simulink model "Spurerkennung"  (R2017a)
settings: Solver=FixedStepDiscrete  StartTime=0.0  StopTime=inf  FixedStep=1/25  RelTol=1e-3  EnableMultiTasking=on
libraries: dspmtrx3 x6, visionanalysis x5, dspvision x2, visionconversions x2, visionsources x1, visionsinks x1
settings Model: NumberOfSteps=5  Creator=Christoph  LastModifiedBy=Christoph
settings SolverCC: EnableConcurrentExecution=on  ConcurrentTasks=on  PositivePriorityOrder=on
settings OptimizationCC: PassReuseOutputArgsAs=Individual arguments  MaxStackSize=64
settings DebuggingCC: ParameterTunabilityLossMsg=error
settings HardwareCC: ProdBitPerPointer=32  ProdBitPerSizeT=32  ProdBitPerPtrDiffT=32  ProdLargestAtomicInteger=Long  ProdLargestAtomicFloat=Double  ProdWordSize=32  ProdHWDeviceType=ARM Compatible->ARM Cortex
settings SFSimCC: MATLABDynamicMemAlloc=off
settings RTWCC: SystemTargetFile=ert.tlc  HardwareBoard=Raspberry Pi  TLCOptions="-aInlineSetEventsForThisBaseRateFcn=TLC_FALSE -aSuppressMultiTaskScheduler=TLC_FALSE  -aRateBasedStepFcn=0"  TemplateMakefile=ert_default_tmf  Description=Embedded Coder  GenerateReport=on  Toolchain=GNU GCC Raspberry Pi  IncludeHyperlinkInReport=on  LaunchReport=on  GenerateTraceInfo=on  GenerateTraceReport=on  GenerateTraceReportSl=on  GenerateTraceReportSf=on  GenerateTraceReportEml=on
settings CodeAppCC: ForceParamTrailComments=on  IgnoreCustomStorageClasses=off  OperatorAnnotations=on  SimulinkDataObjDesc=on  SFDataObjDesc=on  MATLABFcnDesc=on  InsertBlockDesc=on  MATLABSourceComments=on
settings ERTTargetCC: SupportVariableSizeSignals=on

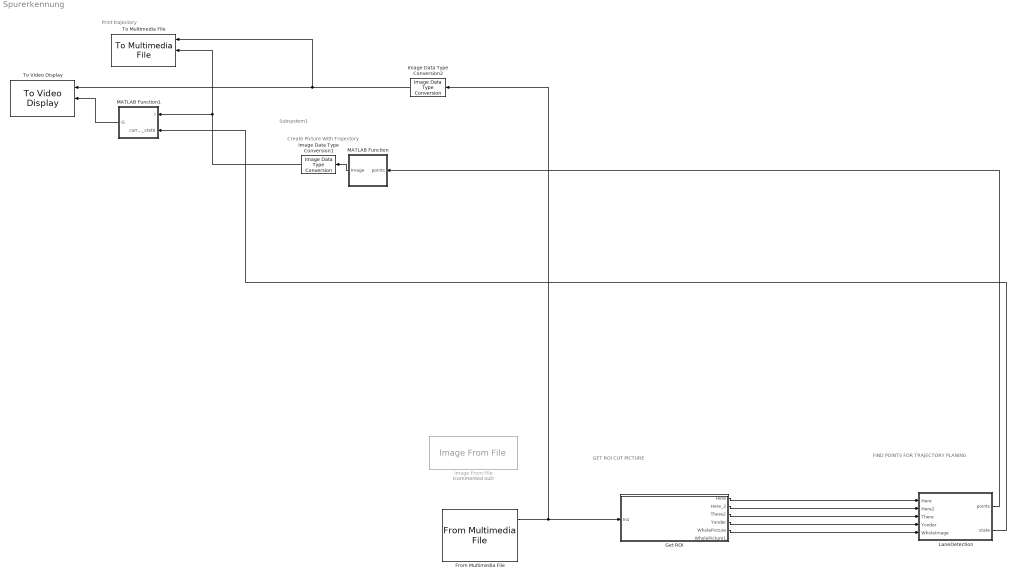
== system Spurerkennung ==
  note: Subsystem1
  note: FIND POINTS FOR TRAJECTORY PLANING
  note: Print trajectory
  note: GET ROI CUT PICTURE
  note: Create Picture With Trajectory
  From Multimedia File : dspvision/From Multimedia File  inputFilename=/Users/Christoph/Documents/workspace/Spurerkennung/Videos/Kreuzung.avi  loop=on  numPlays=inf  outputStreams=Video only  videoDataType=Inherit from file  audioDataType=int16  inheritSampleTime=off  userDefinedSampleTime=1/25  noAudioOutput=off  isIntensityVideo=off  fourcc=RGB  colorVideoFormat=Separate color signals  outputEOF=off  dataOrg=Column-major  audioFrameSize=1024  computeAudioFrameSize=off  outSamplingMode=Sample based
      settings: SourceProductBaseCode=VP
  "Get ROI " : Subsystem
  Image Data Type Conversion1 : visionconversions/Image Data Type Conversion  outDT=single  isSigned=on  wordLen=16  numFracBits=0
      settings: SourceProductName=Computer Vision System Toolbox  SourceProductBaseCode=VP
  Image Data Type Conversion2 : visionconversions/Image Data Type Conversion  outDT=single  isSigned=on  wordLen=16  numFracBits=0
      settings: SourceProductName=Computer Vision System Toolbox  SourceProductBaseCode=VP
  Image From File : visionsources/Image From File  Tag=vipblks_nd  Commented=on  FileName=peppers.png  imagePorts=One multidimensional signal  Ts=inf  ImageDataType=Inherit from input image  Signed=on  WordLength=16  sdImageDataType=uint(8)  FractionLengthMode=User-defined  FractionLength=15  OutPortLabels=R|G|B
      settings: SourceProductName=Computer Vision System Toolbox
  LaneDetection : MATLAB Function  TreatAsAtomicUnit=on
  MATLAB Function : MATLAB Function  TreatAsAtomicUnit=on
  MATLAB Function1 : MATLAB Function  TreatAsAtomicUnit=on
  To Multimedia File : dspvision/To Multimedia File  outputFilename=output.avi  streamSelection=Video only  videoCompressor=None (uncompressed)  audioCompressor=None (uncompressed)  imagePorts=Separate color signals  fileType=AVI  audioDatatype=Determine from input data type  fourcc=RGB  videoQuality=75  mj2000CompFactor=10
      settings: SourceProductName=Computer Vision System Toolbox  SourceProductBaseCode=VP
  To Video Display : visionsinks/To Video Display  windowSizeMode=True size (1:1)  openAtMdlStart=on  fullScreen=off  videoWindowX=547  videoWindowY=164  saveWindowSize=off  videoWindowWidth=640  videoWindowHeight=480  inputColorFormat=RGB  inputType=Obsolete  imagePorts=Separate color signals  OutputDevice=On-screen video monitor  dataOrg=Column-major  isWindowOpen=off
      settings: SourceProductName=Computer Vision System Toolbox
  wires:
  "Get ROI "/1(Here) -> LaneDetection/1(Here)
  "Get ROI "/4(Yonder) -> LaneDetection/4(Yonder)
  Image Data Type Conversion1/1 -> MATLAB Function1/1(I), To Multimedia File/2
  "Get ROI "/3(There2) -> LaneDetection/3(There)
  "Get ROI "/2(Here_2) -> LaneDetection/2(Here2)
  MATLAB Function/1(Image) -> Image Data Type Conversion1/1
  "Get ROI "/5(WholePicture) -> LaneDetection/5(WholeImage)
  Image Data Type Conversion2/1 -> To Multimedia File/1, To Video Display/1
  LaneDetection/1(points) -> MATLAB Function/1(points)
  LaneDetection/2(state) -> MATLAB Function1/2(current_state)
  MATLAB Function1/1(G) -> To Video Display/2
  From Multimedia File/1 -> Image Data Type Conversion2/1, "Get ROI "/1(In1)

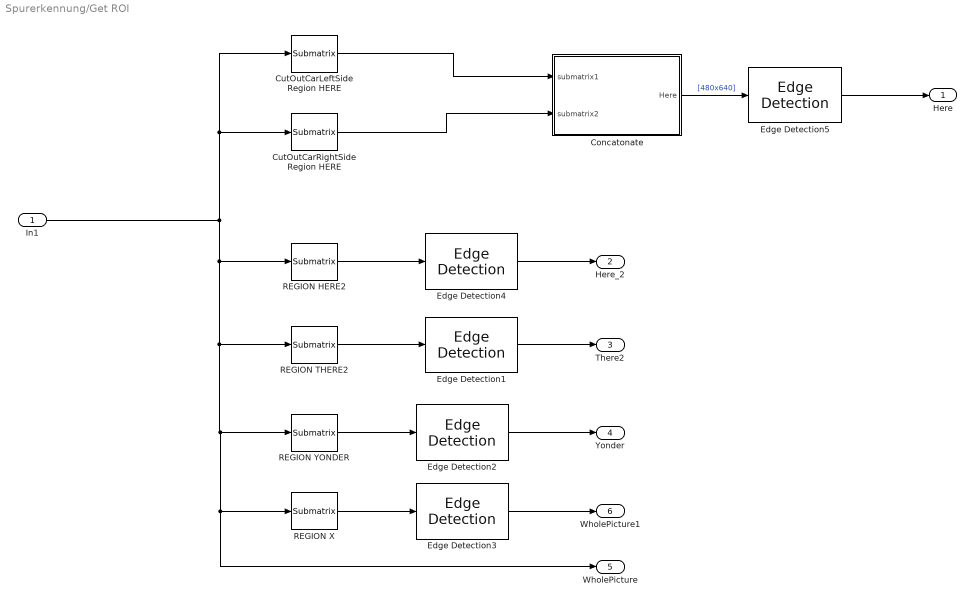
== system Spurerkennung/Get ROI  ==
  In1 : Inport
  Concatonate : MATLAB Function  TreatAsAtomicUnit=on
  CutOutCarLeftSide Region HERE : dspmtrx3/Submatrix  RowSpan=Range of rows  RowStartMode=Index  RowStartIndex=475  RowEndMode=Index  RowEndIndex=480  ColSpan=Range of columns  ColStartMode=Index  ColStartIndex=1  ColEndMode=Index  ColEndIndex=140
  CutOutCarRightSide Region HERE : dspmtrx3/Submatrix  RowSpan=Range of rows  RowStartMode=Index  RowStartIndex=475  RowEndMode=Index  RowEndIndex=480  ColSpan=Range of columns  ColStartMode=Index  ColStartIndex=490  ColEndMode=Last  ColEndIndex=640
  Edge Detection{1..5} (5 alike) : visionanalysis/Edge Detection  method=Sobel  outputType=Binary image  userDefinedThreshold=on  thresholdSource=Specify via dialog  threshold=25  thresholdTuning=4  edgeThinning=off  threshold_canny=[0.1 0.60]  autoPercent=70  sigma=1  prodOutputMode=Binary point scaling  prodOutputWordLength=16  prodOutputFracLength=0  roundingMode=Floor  overflowMode=off
      settings: SourceProductName=Computer Vision System Toolbox  SourceProductBaseCode=VP
  REGION HERE2 : dspmtrx3/Submatrix  RowSpan=Range of rows  RowStartMode=Index  RowStartIndex=330  RowEndMode=Index  RowEndIndex=335  ColSpan=Range of columns  ColStartMode=First  ColStartIndex=1  ColEndMode=Last  ColEndIndex=1
  REGION THERE2 : dspmtrx3/Submatrix  RowSpan=Range of rows  RowStartMode=Index  RowStartIndex=205  RowEndMode=Index  RowEndIndex=210  ColSpan=Range of columns  ColStartMode=First  ColStartIndex=1  ColEndMode=Last  ColEndIndex=1
  REGION X : dspmtrx3/Submatrix  RowSpan=Range of rows  RowStartMode=Index  RowStartIndex=130  RowEndMode=Index  RowEndIndex=135  ColSpan=Range of columns  ColStartMode=First  ColStartIndex=1  ColEndMode=Last  ColEndIndex=1
  REGION YONDER : dspmtrx3/Submatrix  RowSpan=Range of rows  RowStartMode=Index  RowStartIndex=170  RowEndMode=Index  RowEndIndex=175  ColSpan=Range of columns  ColStartMode=First  ColStartIndex=1  ColEndMode=Last  ColEndIndex=1
  Here : Outport
  Here_2 : Outport  Port=2
  There2 : Outport  Port=3
  Yonder : Outport  Port=4
  WholePicture : Outport  Port=5
  WholePicture1 : Outport  Port=6
  wires:
  CutOutCarLeftSide Region HERE/1 -> Concatonate/1(submatrix1)
  In1/1 -> REGION X/1, WholePicture/1, REGION YONDER/1, REGION THERE2/1, REGION HERE2/1, CutOutCarRightSide Region HERE/1, CutOutCarLeftSide Region HERE/1
  CutOutCarRightSide Region HERE/1 -> Concatonate/2(submatrix2)
  REGION HERE2/1 -> Edge Detection4/1
  Edge Detection4/1 -> Here_2/1
  REGION THERE2/1 -> Edge Detection1/1
  Edge Detection1/1 -> There2/1
  REGION YONDER/1 -> Edge Detection2/1
  Edge Detection5/1 -> Here/1
  Concatonate/1(Here) -> Edge Detection5/1  "[480x640]"
  Edge Detection2/1 -> Yonder/1
  REGION X/1 -> Edge Detection3/1
  Edge Detection3/1 -> WholePicture1/1

== matlab function Spurerkennung/MATLAB Function1 ==
  data: I input; G output; current_state input
function G = fcn(I, current_state)

if current_state == 1
    string = 'NORMAL';  
elseif current_state == 2
    string = 'CROSSWALK';  
elseif current_state == 3
    string = 'JUNCTION';

else
    string = 'Normal';
end
    RGB = insertText(I,[1 1],string,'FontSize',18);
G = RGB(:,:,2);

== matlab function Spurerkennung/MATLAB Function ==
  data: Image output; points input
function Image = fcn(points)

%Create picture not necessary if no visualization needed
%TrajectoryImage = zeros(480, 640);

REGIONS_BEGIN = [475 330 205 170];

Image = zeros(480, 640);


for i = 1:size(REGIONS_BEGIN,2)
    Image(REGIONS_BEGIN(i)+2,:) = 1;
end

% 
% p = polyfit(points(1,:), points(2,:), 1);
% x1 = points(1,1);
% x2 = points(1,end);
% x = linspace(x1, x2);
% f = polyval(p,x);
% 
% length_x = size(x,2);
% for j = 1:length_x
%     x_1 = round(x(j));
%     y_1 = round(f(j));
%     if( x_1 >0 && y_1 > 0  && y_1 < 480)
%         Image(y_1, x_1) = 1;
%     end
% end



%disp(points)

lenght = size(points, 2);
% hold off
for i=1:lenght-1
    x1 = points(1,i);
    x2 = points(1,i+1);
    y1 = points(2,i);
    y2 = points(2,i+1);
    p = polyfit([x1 x2], [y1 y2], 1);
%     if(x1 < x2)
%         x2 = 640;
%     else
%         x2 = x2 - 100;
%     end
%     
    x = linspace(x1, x2);
    f = polyval(p, x);
    
    
    length_x = size(x,2);
    for j = 1:length_x
        x_1 = round(x(j));
        y_1 = round(f(j));
        if( x_1 >0 && y_1 > 0  && y_1 < 480)
        Image(y_1, x_1) = 1;
        end
    end
        
        
end

== matlab function Spurerkennung/LaneDetection ==
  data: Here input; Here2 input; There input; Yonder input; WholeImage input; points output; state output

%%%%%%%%% MAIN %%%%%%%%%%%%%%%%%%%%%%%%%%%%%%%%%%%%%%%%%
function [points, state] = fcn(Here, Here2, There, Yonder, WholeImage)

persistent variables
persistent states
persistent initialized
REGIONS = zeros([size(Here) 4]);
REGIONS(:,:,1) = Here;
REGIONS(:,:,2) = Here2;
REGIONS(:,:,3) = There;
REGIONS(:,:,4) = Yonder;

%%%%%%%%%%%%% INIT %%%%%%%%%%%%%%%%%
if(isempty(initialized))
    [variables, states, initialized] = init();
end

%%%%%%%%%%% Sample input %%%%%%%%%%%%%%%%%%%
[all_points, number_of_points]  = FindPointsInLinesAll(variables, REGIONS, true, true);

%%%%%%%%%%%% State machine %%%%%%%%%%%%%%%%%%
[all_points, variables] = RunStateMachine(all_points, number_of_points, WholeImage, states, variables);

points = variables.points_last_found;
state = variables.current_state;
end




%%%%%%%%%%%%%%%%%%%%% State NORMAL %%%%%%%%%%%%%%%%%%%%%%%%%%%%%%%%%%%%%%%%
function [all_points, variables] = StateNormal(all_points, no_points, WholeImage, states, variables)

% Set last state
if variables.current_state ~= variables.last_state
    variables.last_state = variables.current_state;
end

% Switch states if necessary
% [crosswalk_detected, where] = CheckCrosswalk(all_points(3, :, :), no_points, variables.NO_REGIONS);
[stopline_detected] = CheckStopline(WholeImage);

% if crosswalk_detected == true
%     variables.current_state = states.CROSSWALK;
%     return;
if stopline_detected == true
    variables.current_state = states.JUNCTION;
    return;
end

% Search window filtering
[all_points] = CheckPosition(all_points, no_points, variables.NO_REGIONS, variables.VARIABLE_MID, variables.norm);
[all_points] = CheckMarkerWidth(all_points, no_points, variables.NO_REGIONS, variables.EXPECTED_MARKER_WIDTH);
[all_points] = CheckLaneWidth(all_points, no_points, variables.NO_REGIONS, variables.EXPECTED_LANE_WIDTH);

% Select points with highest probabilities
[sel_points, found]  = GetPoints(all_points, no_points, variables.NO_REGIONS);

% Low pass filter
[points_last_found, counter] = LowPassFilter(sel_points, found, variables.points_last_found, variables.counter,...
    variables.NO_REGIONS, variables.MAX_DISTANCES, variables.MAX_COUNTER);
variables.points_last_found = points_last_found;
variables.counter = counter;
end


%%%%%%%%%%%%%%%%%%%%% State Junction %%%%%%%%%%%%%%%%%%%%%%%%%%%%%%%%%%%%%%%%
function [all_points, variables] = StateJunction(all_points, no_points, WholeImage, states, variables)
% This state implemenets a junction specific behavior for lane detection


% Set last state
if variables.current_state ~= variables.last_state
    variables.last_state = variables.current_state;
end

% Switch states if necessary
% [crosswalk_detected, where] = CheckCrosswalk(all_points(3, :, :), no_points, variables.NO_REGIONS);



% Search window filtering % TODO implement more logic for search window
[all_points] = CheckPosition(all_points, no_points, variables.NO_REGIONS, variables.VARIABLE_MID, variables.norm);
[all_points] = CheckMarkerWidth(all_points, no_points, variables.NO_REGIONS, variables.EXPECTED_MARKER_WIDTH);
[all_points] = CheckLaneWidth(all_points, no_points, variables.NO_REGIONS, variables.EXPECTED_LANE_WIDTH);

% Select points with highest probabilities
[sel_points, found]  = GetPoints(all_points, no_points, variables.NO_REGIONS);


% This is the only difference to state normal
MAX_DISTANCES = [10 2 2 10];
[points_last_found, counter] = LowPassFilter(sel_points, found, variables.points_last_found,...
    variables.counter, variables.NO_REGIONS, MAX_DISTANCES, variables.MAX_COUNTER);


[normal_detected] = CheckNormal(points_last_found);

% if crosswalk_detected == true
%     variables.current_state = states.CROSSWALK;
%     return
%     
if normal_detected == true
    variables.current_state = states.NORMAL;
    return;
end

end


%%%%%%%%%%%%%%%%%%%%% State Crosswalk %%%%%%%%%%%%%%%%%%%%%%%%%%%%%%%%%%%%%%%%
function [all_points, variables] = StateCrosswalk(all_points, no_points, WholeImage, states, variables)
% This state implements a crosswalk specific behavior for lane detection

% Set last state
if variables.current_state ~= variables.last_state
    variables.last_state = variables.current_state;
end

points_last_found_temp = variables.points_last_found;
% Switch states if necessary
[crosswalk_detected, where] = CheckCrosswalk(all_points(3, :, :), no_points, variables.NO_REGIONS);

if crosswalk_detected == false
    variables.current_state = states.NORMAL;
    return
end

% Search window filtering % TODO implement more logic for search window
[all_points] = CheckPosition(all_points, no_points, variables.NO_REGIONS, variables.VARIABLE_MID, variables.norm);
[all_points] = CheckMarkerWidth(all_points, no_points, variables.NO_REGIONS, variables.EXPECTED_MARKER_WIDTH);
[all_points] = CheckLaneWidth(all_points, no_points, variables.NO_REGIONS, variables.EXPECTED_LANE_WIDTH);


for REGION = 1:variables.NO_REGIONS
    
    if(where(REGION) == true)
        variables.delay_counter(REGION) = 1;
        variables.points_last_found(:,REGION) = points_last_found_temp(:,REGION);
        
        if (REGION > 1)
            variables.points_last_found(:,REGION-1) = points_last_found_temp(:,REGION-1);
        end
        
    elseif(variables.delay_counter(REGION) >= 0)
        variables.delay_counter(REGION) = variables.delay_counter(REGION) - 1;
        variables.points_last_found(:,REGION) = points_last_found_temp(:,REGION);
        if (REGION > 1)
            variables.points_last_found(:,REGION-1) = points_last_found_temp(:,REGION-1);
        end
    end
end
end


%%%%%%%%%%%%%%%% State machine %%%%%%%%%%%%%%%%%%%%%%%%%%%%%%%%%%%%%%%%%%%
function [all_points, variables] = RunStateMachine(all_points, no_points, WholeImage, states, variables)
% This function is the heart of the state machine

remember_state = 0;

while(remember_state ~= variables.current_state)
    
    if (variables.current_state == states.NORMAL)
        [all_points, variables] = StateNormal(all_points, no_points, WholeImage, states, variables);
        
    elseif (variables.current_state == states.CROSSWALK)
        [all_points, variables] = StateCrosswalk(all_points, no_points, WholeImage, states, variables);
     
    elseif (variables.current_state == states.JUNCTION)
        [all_points, variables] = StateJunction(all_points, no_points, WholeImage, states, variables);
        
    end
    
    remember_state = variables.last_state;
end
end

== matlab function Spurerkennung/Get ROI /Concatonate ==
  data: submatrix1 input; Here output; submatrix2 input
function Here  = fcn(submatrix1, submatrix2)
% This function supposed to create a new image with just the Points of
% interests (Region of Interest)

% Region Here
Here = zeros(6,640);

%Cut out car and Region HERE
Here(1:6,1:140) = submatrix1;
Here(1:6,490:640) = submatrix2;
